simulink library "send_b"  (R2024b)
settings: Solver=VariableStepAuto  StartTime=0.0  StopTime=10.0  RelTol=1e-3
settings Model: Creator=eikel  LastModifiedBy=eikel

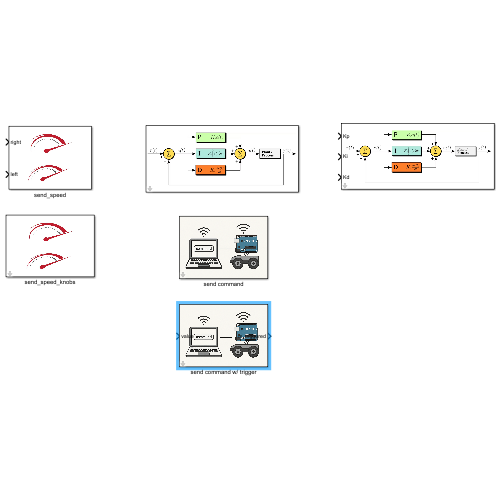
[thumbnail: Simulink's stored preview of the top-level diagram]
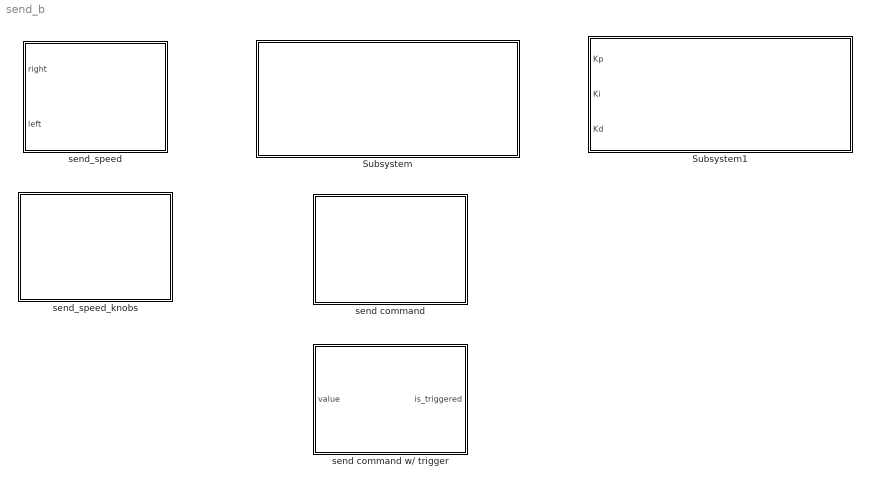
== system send_b ==
  Subsystem : Subsystem  mask{kp=0, ki=0, kd=0}
      mask Display: image('PID.png', [0,0,0,0,100,80]);
  Subsystem1 : Subsystem
      mask Display: image('PID.png', [0,0,0,0,100,80]);
  send command : Subsystem  mask{cmd=start}
      mask prompts: cmd "command"
      mask TypeOptions cmd: start | stop | pid-mode
      mask Display: image('command.png');
  send command w/ trigger : Subsystem
      mask Display: image('command.png');
  send_speed : Subsystem
      mask Display: image('speed.jpg');
  send_speed_knobs : Subsystem  mask{left=-8.0, right=0}
      mask prompts: left "left speed"; right "right speed"
      mask Display: image('speed.jpg');

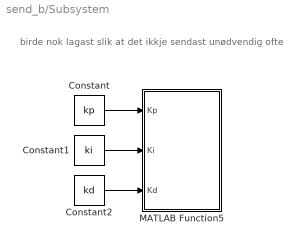
== system send_b/Subsystem ==
  note: birde nok lagast slik at det ikkje sendast unødvendig ofte
  Constant : Constant  Value=kp
  Constant1 : Constant  Value=ki
  Constant2 : Constant  Value=kd
  MATLAB Function5 : MATLAB Function  TreatAsAtomicUnit=on
  wires:
  Constant1/1 -> MATLAB Function5/2(Ki)
  Constant/1 -> MATLAB Function5/1(Kp)
  Constant2/1 -> MATLAB Function5/3(Kd)

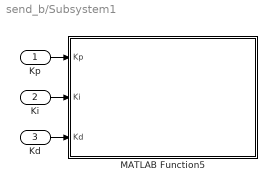
== system send_b/Subsystem1 ==
  Kp : Inport
  Ki : Inport  Port=2
  Kd : Inport  Port=3
  MATLAB Function5 : MATLAB Function  TreatAsAtomicUnit=on
  wires:
  Kp/1 -> MATLAB Function5/1(Kp)
  Ki/1 -> MATLAB Function5/2(Ki)
  Kd/1 -> MATLAB Function5/3(Kd)

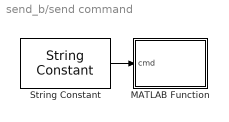
== system send_b/send command ==
  MATLAB Function : MATLAB Function  TreatAsAtomicUnit=on
  String Constant : StringConstant  String=cmd
  wires:
  String Constant/1 -> MATLAB Function/1(cmd)

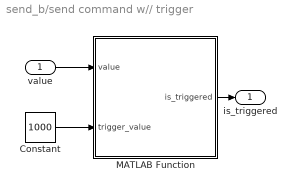
== system send_b/send command w// trigger ==
  value : Inport
  Constant : Constant  Value=1000
  MATLAB Function : MATLAB Function  TreatAsAtomicUnit=on
  is_triggered : Outport
  wires:
  MATLAB Function/1(is_triggered) -> is_triggered/1
  value/1 -> MATLAB Function/1(value)
  Constant/1 -> MATLAB Function/2(trigger_value)

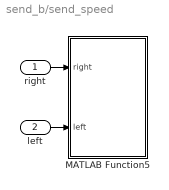
== system send_b/send_speed ==
  right : Inport
  left : Inport  Port=2
  MATLAB Function5 : MATLAB Function  TreatAsAtomicUnit=on
  wires:
  left/1 -> MATLAB Function5/2(left)
  right/1 -> MATLAB Function5/1(right)

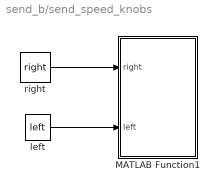
== system send_b/send_speed_knobs ==
  MATLAB Function1 : MATLAB Function  TreatAsAtomicUnit=on
  left : Constant  Value=left
  right : Constant  Value=right
  wires:
  left/1 -> MATLAB Function1/2(left)
  right/1 -> MATLAB Function1/1(right)

== matlab function send_b/Subsystem/MATLAB Function5 ==
  data: Kp input; Ki input; Kd input
function publish_PID(Kp, Ki, Kd)
    coder.extrinsic('send_PID');  

    persistent last_Kp last_Ki last_Kd

    if isempty(last_Kp)
        last_Kp = NaN; % sørg for første utsending
        last_Ki = NaN;
        last_Kd = NaN;
    end

    % Sjekk om noko har endra seg
    if Kp ~= last_Kp || Ki ~= last_Ki || Kd ~= last_Kd
        send_PID(Kp, Ki, Kd); % send berre om noko endra seg
        last_Kp = Kp;
        last_Ki = Ki;
        last_Kd = Kd;
    end
end

== matlab function send_b/send_speed_knobs/MATLAB Function1 ==
  data: right input; left input
function publish_speed(right, left)
    coder.extrinsic('send_speed');  % kallar på ekstern MATLAB-funksjon

    persistent last_right last_left

    if isempty(last_right)
        last_right = NaN;
        last_left  = NaN;
    end

    if right ~= last_right || left ~= last_left
        send_speed(right, left); % berre send om verdiar har endra seg
        last_right = right;
        last_left  = left;
    end
end

== matlab function send_b/send command/MATLAB Function ==
  data: cmd input
function publish_cmd(cmd)
    coder.extrinsic('send_cmd');

    persistent last_cmd
    if isempty(last_cmd)
        last_cmd = blanks(20);  % 1x20 char-array
    end

    % Konverter input til char
    cmd_char = char(cmd);
    L = length(cmd_char);

    % Sørg for at cmd_padded er ALLTID 1x20
    cmd_padded = blanks(20);      % Alloker fast lengde
    N = min(L, 20);               % maks 20 teikn
    cmd_padded(1:N) = cmd_char(1:N);  % kopier teikna

    % Samanlikn og send berre ved endring
    if ~strcmp(cmd_padded, last_cmd)
        send_cmd(strtrim(cmd_padded));  % send utan whitespace
        last_cmd = cmd_padded;          % lagre nytt for samanlikning
    end
end

== matlab function send_b/send command w// trigger/MATLAB Function ==
  settings: updateMethod=DISCRETE  sampleTime=0.1
  data: value input; trigger_value input; is_triggered output
function is_triggered = publish_cmd_trigger(value, trigger_value)
    coder.extrinsic('send_cmd');

    persistent last_cmd
    if isempty(last_cmd)
        last_cmd = 0;  % tom int
    end

    

    if value > trigger_value
        is_triggered = true;
        cmd = 1;
    else
        is_triggered = false;
        cmd = 0;
    end

    if cmd ~= last_cmd
        send_cmd(cmd);
        last_cmd = cmd;
    end
end

== matlab function send_b/Subsystem1/MATLAB Function5 ==
  data: Kp input; Ki input; Kd input
function publish_PID(Kp, Ki, Kd)
    coder.extrinsic('send_PID');  

    persistent last_Kp last_Ki last_Kd

    if isempty(last_Kp)
        last_Kp = NaN; % sørg for første utsending
        last_Ki = NaN;
        last_Kd = NaN;
    end

    % Sjekk om noko har endra seg
    if Kp ~= last_Kp || Ki ~= last_Ki || Kd ~= last_Kd
        send_PID(Kp, Ki, Kd); % send berre om noko endra seg
        last_Kp = Kp;
        last_Ki = Ki;
        last_Kd = Kd;
    end
end

== matlab function send_b/send_speed/MATLAB Function5 ==
  data: right input; left input
function publish_speed(right, left)
    coder.extrinsic('send_speed');  % merk: dette peikar på .m-fila di
    send_speed(right, left)
end
